simulink model "magball"  (R2020b)
settings: Solver=VariableStepAuto  StartTime=0.0  StopTime=10.0  RelTol=1e-3
settings Model: Creator=duzun  LastModifiedBy=duzun

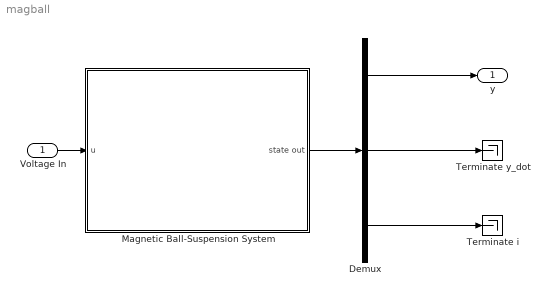
== system magball ==
  Voltage In : Inport
  Demux : Demux  Outputs=3
  Magnetic Ball-Suspension System : Subsystem
  Terminate i : Terminator
  Terminate y_dot : Terminator
  y : Outport
  wires:
  Voltage In/1 -> Magnetic Ball-Suspension System/1(u)
  Magnetic Ball-Suspension System/1(state out) -> Demux/1
  Demux/1 -> y/1
  Demux/2 -> Terminate y_dot/1
  Demux/3 -> Terminate i/1

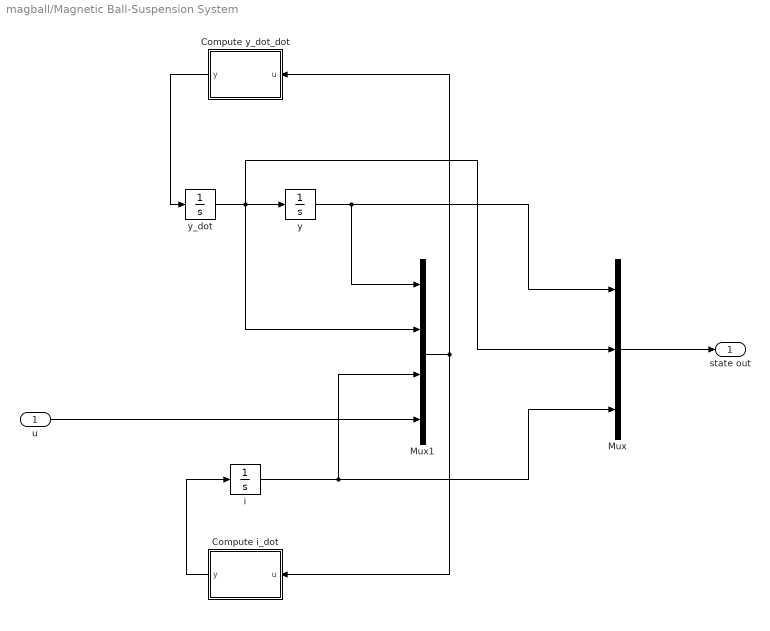
== system magball/Magnetic Ball-Suspension System ==
  u : Inport
  Compute i_dot : MATLAB Function  TreatAsAtomicUnit=on
  Compute y_dot_dot : MATLAB Function  TreatAsAtomicUnit=on
  Mux : Mux  Inputs=3
  Mux1 : Mux
  i : Integrator
  y : Integrator
  y_dot : Integrator
  state out : Outport
  wires:
  Mux/1 -> state out/1
  y_dot/1 -> Mux1/2, Mux/2, y/1
  y/1 -> Mux1/1, Mux/1
  i/1 -> Mux1/3, Mux/3
  u/1 -> Mux1/4
  Mux1/1 -> Compute i_dot/1(u), Compute y_dot_dot/1(u)
  Compute y_dot_dot/1(y) -> y_dot/1
  Compute i_dot/1(y) -> i/1

== matlab function magball/Magnetic Ball-Suspension System/Compute y_dot_dot ==
  data: u input; y output
function y = fcn(u)
y = 9.8-(u(3)^2)/(u(1)^2);

== matlab function magball/Magnetic Ball-Suspension System/Compute i_dot ==
  data: u input; y output
function y = fcn(u)
y = u(4)-3*u(3);
